simulink model "RasPiTCP_LedCtrl"  (R2018a)
settings: Solver=FixedStepAuto  StartTime=0.0  StopTime=inf  RelTol=1e-3  EnableMultiTasking=on
PreLoadFcn:
  | RasPiTcpConfig;
  | RasPiTcpDataType;
values from neighbouring files (symbols this model uses):
  LedInValidCommandMessage = 'Invalid Command'    [RasPiTcpConfig.m]
  LedOffMessage = "L.E.D is OFF   "    [RasPiTcpConfig.m]
  LedOnMessage = 'L.E.D is ON    '    [RasPiTcpConfig.m]
  TcpBufferInit = zeros(1,TcpBufferSize)    [RasPiTcpConfig.m]
undefined symbols (not defined in the file or in its folder): Green, led0, LedStatus
libraries: simulink x5, raspberrypilib x2, embdlinuxlib x2
settings Model: SimulationMode=external  Creator=swararag  LastModifiedBy=swararag
settings SolverCC: PositivePriorityOrder=on
settings OptimizationCC: EnhancedBackFolding=on  PassReuseOutputArgsAs=Individual arguments  MaxStackSize=64  OptimizeBlockOrder=speed  DifferentSizesBufferReuse=on  OptimizationCustomize=off
settings DebuggingCC: ParameterTunabilityLossMsg=error
settings HardwareCC: ProdBitPerPointer=32  ProdBitPerSizeT=32  ProdBitPerPtrDiffT=32  ProdLargestAtomicInteger=Long  ProdLargestAtomicFloat=Double  ProdWordSize=32  ProdHWDeviceType=ARM Compatible->ARM Cortex
settings SFSimCC: MATLABDynamicMemAlloc=off
settings RTWCC: SystemTargetFile=ert.tlc  HardwareBoard=Raspberry Pi  TLCOptions="-aInlineSetEventsForThisBaseRateFcn=TLC_FALSE -aSuppressMultiTaskScheduler=TLC_FALSE  -aRateBasedStepFcn=0"  TemplateMakefile=ert_default_tmf  GenerateReport=on  Toolchain=GNU GCC Raspberry Pi  BuildConfiguration=Faster Runs  IncludeHyperlinkInReport=on  LaunchReport=on  GenerateTraceInfo=on  GenerateTraceReport=on  GenerateTraceReportSl=on  GenerateTraceReportSf=on  GenerateTraceReportEml=on
settings CodeAppCC: ForceParamTrailComments=on  IgnoreCustomStorageClasses=off  OperatorAnnotations=on  SimulinkDataObjDesc=on  SFDataObjDesc=on  InsertBlockDesc=on
settings ERTTargetCC: SupportVariableSizeSignals=on  GenerateASAP2=on  ERTFilePackagingFormat=Compact

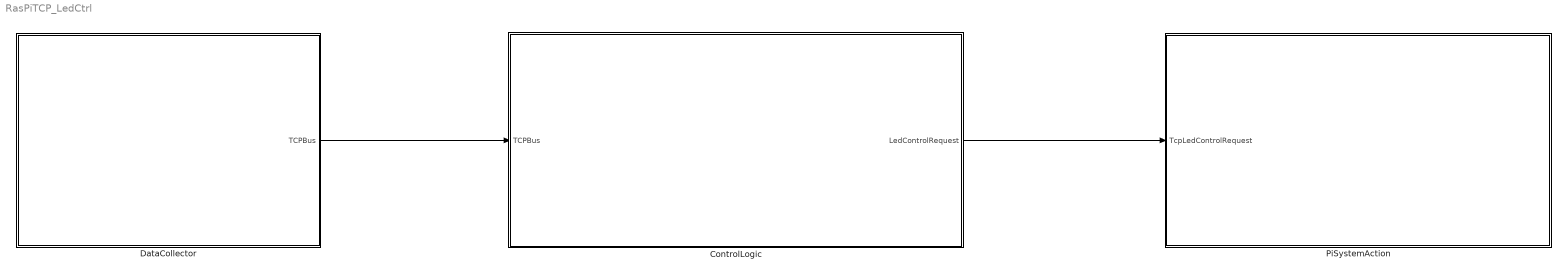
== system RasPiTCP_LedCtrl ==
  ControlLogic : Subsystem  Priority=1  TreatAsAtomicUnit=on
      settings: RTWFcnNameOpts=Use subsystem name
  DataCollector : Subsystem  Priority=0  TreatAsAtomicUnit=on
      settings: RTWFcnNameOpts=Use subsystem name
  PiSystemAction : Subsystem  Priority=2  TreatAsAtomicUnit=on
      settings: RTWFcnNameOpts=Use subsystem name  FunctionWithSeparateData=on
  wires:
  DataCollector/1(TCPBus) -> ControlLogic/1(TCPBus)
  ControlLogic/1(LedControlRequest) -> PiSystemAction/1(TcpLedControlRequest)

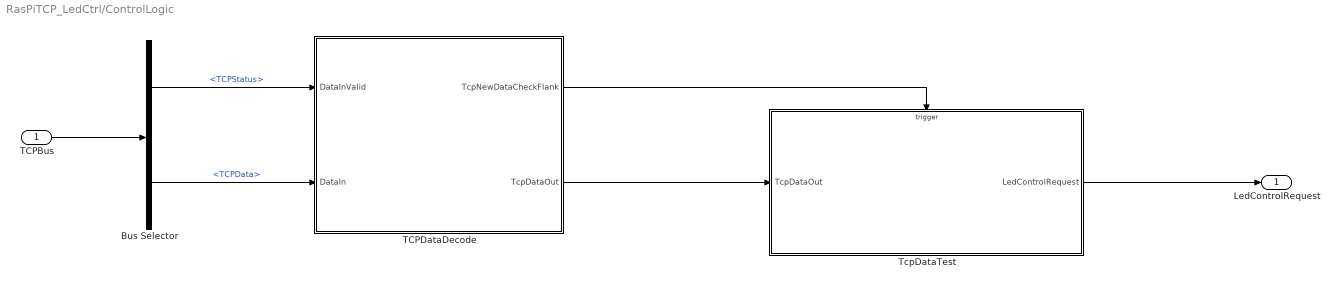
== system RasPiTCP_LedCtrl/ControlLogic ==
  TCPBus : Inport
  Bus Selector : BusSelector  OutputSignals=TCPStatus,TCPData
  TCPDataDecode : Subsystem  TreatAsAtomicUnit=on
  TcpDataTest : Subsystem
  LedControlRequest : Outport
  wires:
  TCPBus/1 -> Bus Selector/1
  Bus Selector/1 -> TCPDataDecode/1(DataInValid)  "<TCPStatus>"
  Bus Selector/2 -> TCPDataDecode/2(DataIn)  "<TCPData>"
  TCPDataDecode/2(TcpDataOut) -> TcpDataTest/1(TcpDataOut)
  TcpDataTest/1(LedControlRequest) -> LedControlRequest/1
  TCPDataDecode/1(TcpNewDataCheckFlank) -> TcpDataTest/Trigger

== system RasPiTCP_LedCtrl/DataCollector ==
  Bus Creator : BusCreator  Inputs=2
  Data Type Conversion : DataTypeConversion  OutDataTypeStr=boolean
  TCP/IP Receive : raspberrypilib/TCP//IP Receive  Mode_=Server  LocalServerPort_=TcpServerRxPort  RemoteAddr_=192.186.0.130  RemoteServerPort_=25001  DataType_=uint8  DataSize_=1  SampleTime_=0.05  SimulateUsing=Code generation  ClientPortBindingSelection_=off  ClientPortToBind_=35000  BlockingMode_=on  BlockTimeout_=TcpServerRxTimeOut
      settings: SourceProductName=Simulink Support Package for Raspberry Pi Hardware  SourceProductBaseCode=RASPPI
  TCPBus : Outport
  wires:
  TCP/IP Receive/2 -> Data Type Conversion/1
  Bus Creator/1 -> TCPBus/1
  Data Type Conversion/1 -> Bus Creator/2  "TCPStatus"
  TCP/IP Receive/1 -> Bus Creator/1  "TCPData"

== system RasPiTCP_LedCtrl/PiSystemAction ==
  TcpLedControlRequest : Inport
  Bus Selector : BusSelector  OutputSignals=LedControlRequestFlank,LedState
  TCPSend : Subsystem
      settings: RTWFcnNameOpts=Use subsystem name
  wires:
  TcpLedControlRequest/1 -> Bus Selector/1
  Bus Selector/2 -> TCPSend/1(LedStatus)  "<LedState>"
  Bus Selector/1 -> TCPSend/Trigger  "<LedControlRequestFlank>"

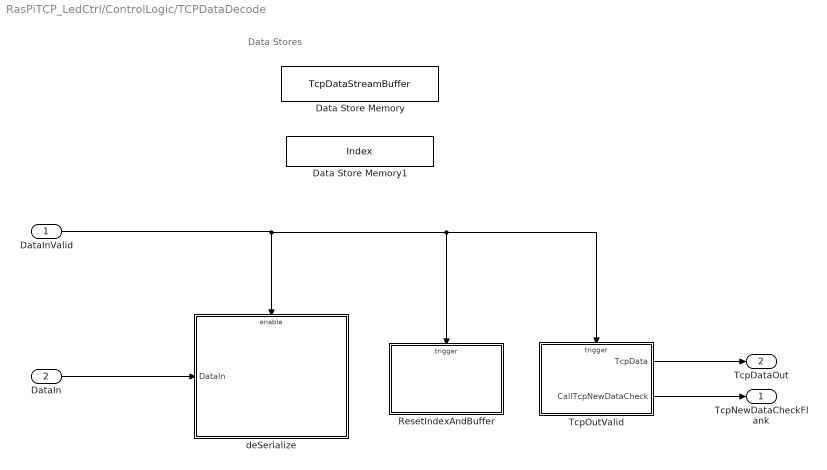
== system RasPiTCP_LedCtrl/ControlLogic/TCPDataDecode ==
  note: Data Stores
  DataInValid : Inport
  DataIn : Inport  Port=2
  Data Store Memory : DataStoreMemory  DataStoreName=TcpDataStreamBuffer  ReadBeforeWriteMsg=warning  WriteAfterWriteMsg=warning  WriteAfterReadMsg=warning  InitialValue=TcpBufferInit  ShowAdditionalParam=off  OutDataTypeStr=uint8
  Data Store Memory1 : DataStoreMemory  DataStoreName=Index  ReadBeforeWriteMsg=warning  WriteAfterWriteMsg=warning  WriteAfterReadMsg=warning  InitialValue=1  ShowAdditionalParam=off  OutDataTypeStr=uint8
  ResetIndexAndBuffer : Subsystem  Priority=0  TreatAsAtomicUnit=on
  TcpOutValid : Subsystem  Priority=1  TreatAsAtomicUnit=on
  deSerialize : Subsystem  Priority=0
  TcpNewDataCheckFlank : Outport
  TcpDataOut : Outport  Port=2
  wires:
  TcpOutValid/1(TcpData) -> TcpDataOut/1
  DataIn/1 -> deSerialize/1(DataIn)
  DataInValid/1 -> deSerialize/Enable, TcpOutValid/Trigger, ResetIndexAndBuffer/Trigger
  TcpOutValid/2(CallTcpNewDataCheck) -> TcpNewDataCheckFlank/1

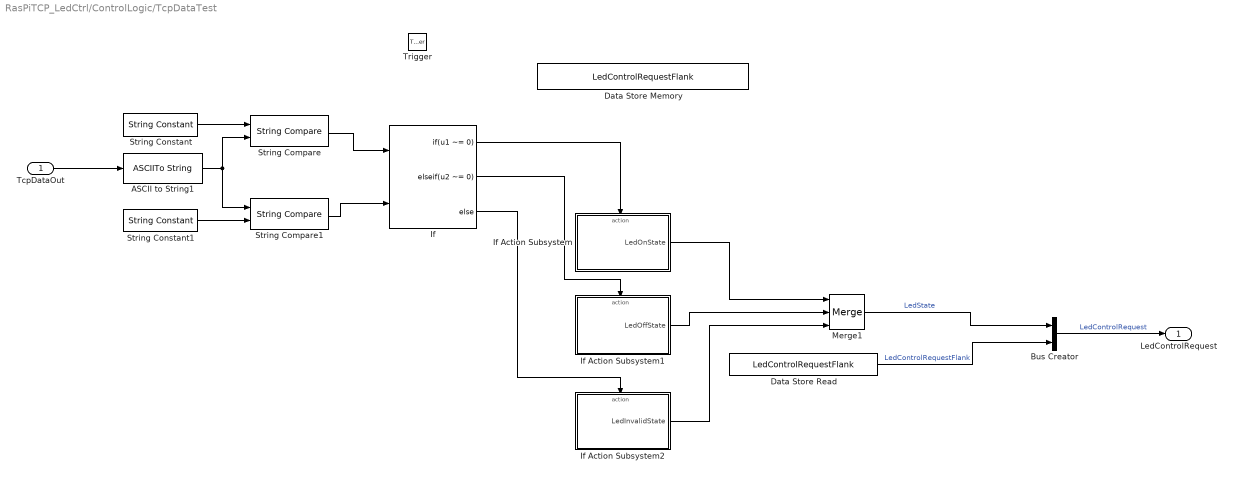
== system RasPiTCP_LedCtrl/ControlLogic/TcpDataTest ==
  TcpDataOut : Inport
  Trigger : TriggerPort  TriggerType=function-call  VariantControl=Variant  InitialTriggerSignalState=zero  PortDimensions=1
  ASCII to String1 : ASCIIToString
  Bus Creator : BusCreator  Inputs=2
  Data Store Memory : DataStoreMemory  DataStoreName=LedControlRequestFlank  ReadBeforeWriteMsg=warning  WriteAfterWriteMsg=warning  WriteAfterReadMsg=warning  InitialValue=1  ShowAdditionalParam=off  OutDataTypeStr=boolean
  Data Store Read : DataStoreRead  DataStoreName=LedControlRequestFlank
  If : If  NumInputs=2  IfExpression=u1 ~= 0  ElseIfExpressions=u2 ~= 0
  If Action Subsystem : Subsystem  TreatAsAtomicUnit=on
  If Action Subsystem1 : Subsystem  TreatAsAtomicUnit=on
  If Action Subsystem2 : Subsystem  TreatAsAtomicUnit=on
  Merge1 : Merge  Inputs=3  InitialOutput=LedStatus.OFF
  String Compare : StringCompare  CaseSensitive=off
  String Compare1 : StringCompare  CaseSensitive=off
  String Constant : StringConstant  String=LedOnText
  String Constant1 : StringConstant  String=LedOffText
  LedControlRequest : Outport
      settings: EnsureOutportIsVirtual=on
  wires:
  If/3 -> If Action Subsystem2/Action
  String Compare1/1 -> If/2
  ASCII to String1/1 -> String Compare1/1, String Compare/2
  If/2 -> If Action Subsystem1/Action
  If/1 -> If Action Subsystem/Action
  String Constant1/1 -> String Compare1/2
  String Constant/1 -> String Compare/1
  String Compare/1 -> If/1
  TcpDataOut/1 -> ASCII to String1/1
  If Action Subsystem2/1(LedInvalidState) -> Merge1/3
  If Action Subsystem1/1(LedOffState) -> Merge1/2
  If Action Subsystem/1(LedOnState) -> Merge1/1
  Merge1/1 -> Bus Creator/1  "LedState"
  Bus Creator/1 -> LedControlRequest/1  "LedControlRequest"
  Data Store Read/1 -> Bus Creator/2  "LedControlRequestFlank"

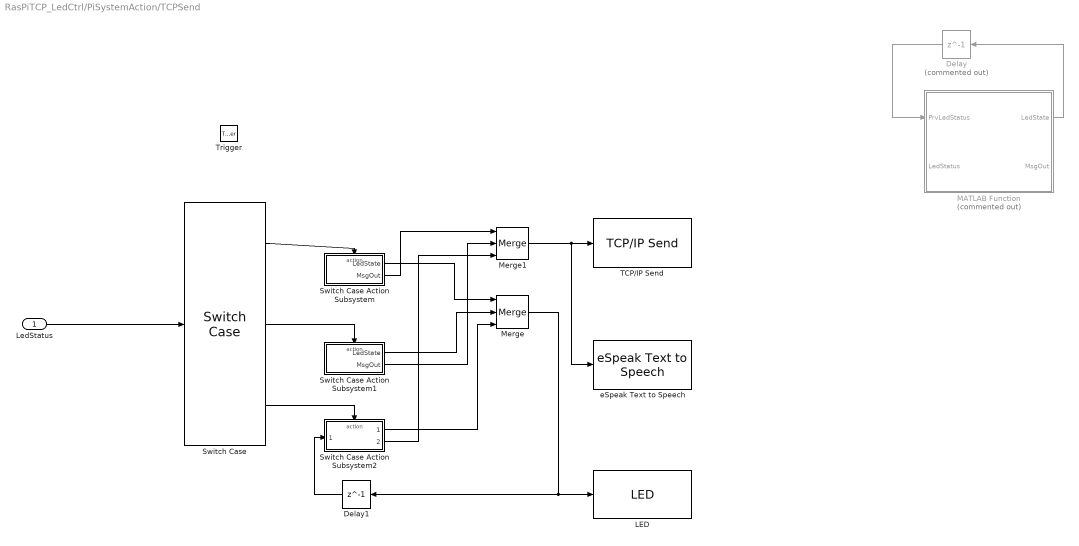
== system RasPiTCP_LedCtrl/PiSystemAction/TCPSend ==
  LedStatus : Inport  OutDataTypeStr=Enum: LedStatus
  Trigger : TriggerPort  TriggerType=either  VariantControl=Variant
  Delay : Delay  Commented=on  DelayLength=1  InitialCondition=false
  Delay1 : Delay  DelayLength=1  InitialCondition=false
  LED : embdlinuxlib/LED  board=Model B+  led=led0 (Green)  blockPlatform=Raspberry Pi
      settings: SourceProductName=Simulink Support Package for Raspberry Pi Hardware  SourceProductBaseCode=RASPPI
  MATLAB Function : MATLAB Function  Commented=on  TreatAsAtomicUnit=on
  Merge : Merge  Inputs=3  InitialOutput=false
  Merge1 : Merge  Inputs=3
  Switch Case : SwitchCase  CaseConditions={LedStatus.ON, LedStatus.OFF}
  Switch Case Action Subsystem : Subsystem  TreatAsAtomicUnit=on
  Switch Case Action Subsystem1 : Subsystem  TreatAsAtomicUnit=on
  Switch Case Action Subsystem2 : Subsystem  TreatAsAtomicUnit=on
  TCP/IP Send : raspberrypilib/TCP//IP Send  Mode_=Server  LocalServerPort_=TcpServerTxPort  RemoteAddr_=192.168.0.117  RemoteServerPort_=25000  SimulateUsing=Code generation  ClientPortBindingSelection_=off  ClientPortToBind_=35000  BlockingMode_=on  BlockTimeout_=TcpServerTxTimeOut
      settings: SourceProductName=Simulink Support Package for Raspberry Pi Hardware  SourceProductBaseCode=RASPPI
  eSpeak Text to Speech : embdlinuxlib/eSpeak Text to Speech  blockPlatform=Raspberry Pi
      settings: SourceProductName=Simulink Support Package for Raspberry Pi Hardware  SourceProductBaseCode=RASPPI
  wires:
  MATLAB Function/1(LedState) -> Delay/1
  Switch Case/1 -> Switch Case Action Subsystem/Action
  Switch Case/2 -> Switch Case Action Subsystem1/Action
  Switch Case Action Subsystem/1(LedState) -> Merge/1
  Switch Case Action Subsystem1/1(LedState) -> Merge/2
  LedStatus/1 -> Switch Case/1
  Delay/1 -> MATLAB Function/1(PrvLedStatus)
  Switch Case/3 -> Switch Case Action Subsystem2/Action
  Switch Case Action Subsystem2/1(LedState) -> Merge/3
  Merge/1 -> Delay1/1, LED/1
  Delay1/1 -> Switch Case Action Subsystem2/1(PrvState)
  Merge1/1 -> eSpeak Text to Speech/1, TCP/IP Send/1
  Switch Case Action Subsystem2/2(MsgOut) -> Merge1/3
  Switch Case Action Subsystem1/2(MsgOut) -> Merge1/2
  Switch Case Action Subsystem/2(MsgOut) -> Merge1/1

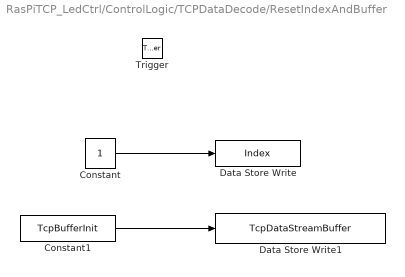
== system RasPiTCP_LedCtrl/ControlLogic/TCPDataDecode/ResetIndexAndBuffer ==
  Trigger : TriggerPort  VariantControl=Variant  InitialTriggerSignalState=zero  PortDimensions=1
  Constant : Constant  OutDataTypeStr=uint8
  Constant1 : Constant  Value=TcpBufferInit  OutDataTypeStr=uint8
  Data Store Write : DataStoreWrite  DataStoreName=Index
  Data Store Write1 : DataStoreWrite  DataStoreName=TcpDataStreamBuffer
  wires:
  Constant/1 -> Data Store Write/1
  Constant1/1 -> Data Store Write1/1

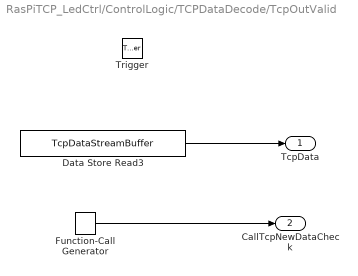
== system RasPiTCP_LedCtrl/ControlLogic/TCPDataDecode/TcpOutValid ==
  Trigger : TriggerPort  TriggerType=falling  VariantControl=Variant  InitialTriggerSignalState=zero  PortDimensions=1
  Data Store Read3 : DataStoreRead  DataStoreName=TcpDataStreamBuffer
  Function-Call Generator : simulink/Ports & Subsystems/Function-Call Generator  sample_time=-1  numberOfIterations=1
  TcpData : Outport
  CallTcpNewDataCheck : Outport  Port=2
  wires:
  Data Store Read3/1 -> TcpData/1
  Function-Call Generator/1 -> CallTcpNewDataCheck/1

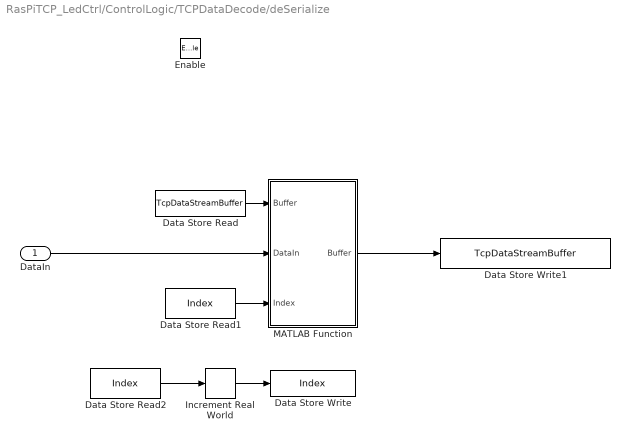
== system RasPiTCP_LedCtrl/ControlLogic/TCPDataDecode/deSerialize ==
  DataIn : Inport
  Enable : EnablePort  PropagateVarSize=During execution
  Data Store Read : DataStoreRead  DataStoreName=TcpDataStreamBuffer
  Data Store Read1 : DataStoreRead  DataStoreName=Index
  Data Store Read2 : DataStoreRead  Priority=8  DataStoreName=Index
  Data Store Write : DataStoreWrite  DataStoreName=Index
  Data Store Write1 : DataStoreWrite  DataStoreName=TcpDataStreamBuffer
  Increment Real World : simulink/Additional Math & Discrete/Additional Math: Increment - Decrement/Increment Real World
      settings: SourceProductName=Simulink  SourceProductBaseCode=SL
  MATLAB Function : MATLAB Function  Priority=1  TreatAsAtomicUnit=on
  wires:
  DataIn/1 -> MATLAB Function/2(DataIn)
  MATLAB Function/1(Buffer) -> Data Store Write1/1
  Data Store Read/1 -> MATLAB Function/1("Buffer ")
  Data Store Read1/1 -> MATLAB Function/3(Index)
  Increment Real World/1 -> Data Store Write/1
  Data Store Read2/1 -> Increment Real World/1

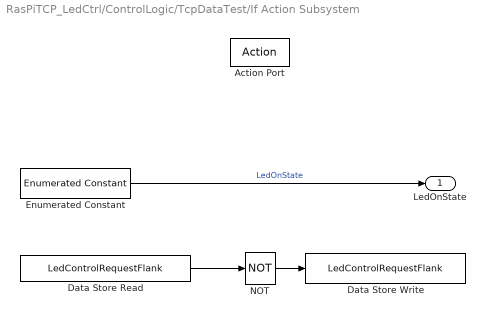
== system RasPiTCP_LedCtrl/ControlLogic/TcpDataTest/If Action Subsystem ==
  Action Port : ActionPort  ActionType=then
  Data Store Read : DataStoreRead  DataStoreName=LedControlRequestFlank
  Data Store Write : DataStoreWrite  DataStoreName=LedControlRequestFlank
  Enumerated Constant : simulink/Sources/Enumerated Constant  OutDataTypeStr=Enum: LedStatus  Value=LedStatus.ON  SampleTime=inf
      settings: SourceProductName=Simulink
  NOT : Logic  Operator=NOT  IconShape=distinctive  AllPortsSameDT=off  OutDataTypeStr=boolean
  LedOnState : Outport
  wires:
  Enumerated Constant/1 -> LedOnState/1  "LedOnState"
  Data Store Read/1 -> NOT/1
  NOT/1 -> Data Store Write/1

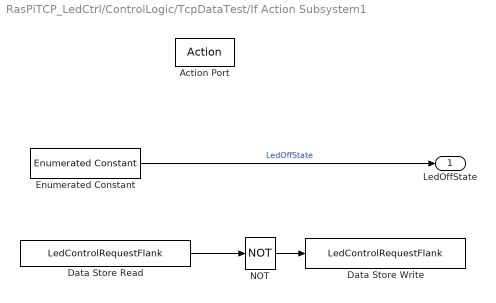
== system RasPiTCP_LedCtrl/ControlLogic/TcpDataTest/If Action Subsystem1 ==
  Action Port : ActionPort  ActionType=elseif
  Data Store Read : DataStoreRead  DataStoreName=LedControlRequestFlank
  Data Store Write : DataStoreWrite  DataStoreName=LedControlRequestFlank
  Enumerated Constant : simulink/Sources/Enumerated Constant  OutDataTypeStr=Enum: LedStatus  Value=LedStatus.OFF  SampleTime=inf
      settings: SourceProductName=Simulink
  NOT : Logic  Operator=NOT  IconShape=distinctive  AllPortsSameDT=off  OutDataTypeStr=boolean
  LedOffState : Outport
  wires:
  Enumerated Constant/1 -> LedOffState/1  "LedOffState"
  Data Store Read/1 -> NOT/1
  NOT/1 -> Data Store Write/1

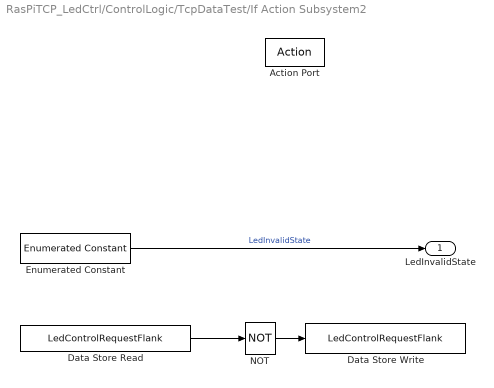
== system RasPiTCP_LedCtrl/ControlLogic/TcpDataTest/If Action Subsystem2 ==
  Action Port : ActionPort  ActionType=else
  Data Store Read : DataStoreRead  DataStoreName=LedControlRequestFlank
  Data Store Write : DataStoreWrite  DataStoreName=LedControlRequestFlank
  Enumerated Constant : simulink/Sources/Enumerated Constant  OutDataTypeStr=Enum: LedStatus  Value=LedStatus.INVALID  SampleTime=inf
      settings: SourceProductName=Simulink
  NOT : Logic  Operator=NOT  IconShape=distinctive  AllPortsSameDT=off  OutDataTypeStr=boolean
  LedInvalidState : Outport
  wires:
  Enumerated Constant/1 -> LedInvalidState/1  "LedInvalidState"
  Data Store Read/1 -> NOT/1
  NOT/1 -> Data Store Write/1

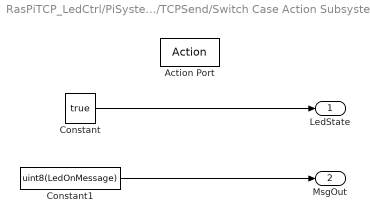
== system RasPiTCP_LedCtrl/PiSystemAction/TCPSend/Switch Case Action Subsystem ==
  Action Port : ActionPort  ActionType=case
  Constant : Constant  Value=true  OutDataTypeStr=boolean
  Constant1 : Constant  Value=uint8(LedOnMessage)  OutDataTypeStr=uint8
  LedState : Outport
  MsgOut : Outport  Port=2
  wires:
  Constant/1 -> LedState/1
  Constant1/1 -> MsgOut/1

== system RasPiTCP_LedCtrl/PiSystemAction/TCPSend/Switch Case Action Subsystem1 ==
  Action Port : ActionPort  ActionType=case
  Constant : Constant  Value=false  OutDataTypeStr=boolean
  Constant1 : Constant  Value=uint8(LedOffMessage)  OutDataTypeStr=uint8
  LedState : Outport
  MsgOut : Outport  Port=2
  wires:
  Constant/1 -> LedState/1
  Constant1/1 -> MsgOut/1

== system RasPiTCP_LedCtrl/PiSystemAction/TCPSend/Switch Case Action Subsystem2 ==
  PrvState : Inport
  Action Port : ActionPort  ActionType=default
  Constant1 : Constant  Value=uint8(LedInValidCommandMessage)  OutDataTypeStr=uint8
  LedState : Outport
  MsgOut : Outport  Port=2
  wires:
  PrvState/1 -> LedState/1
  Constant1/1 -> MsgOut/1

== matlab function RasPiTCP_LedCtrl/ControlLogic/TCPDataDecode/deSerialize/MATLAB Function ==
  data: Buffer input; DataIn input; Index input; Buffer output
function Buffer =fcn(Buffer,DataIn,Index)


Buffer(Index)=DataIn;


end

== matlab function RasPiTCP_LedCtrl/PiSystemAction/TCPSend/MATLAB Function ==
  data: PrvLedStatus input; LedStatus input; LedState output; MsgOut output
function [LedState,MsgOut]= fcn(PrvLedStatus,LedStatus)

switch LedStatus
   case OFF
        LedState = false; 
        MsgOut = uint8('L.E.D is OFF   ');
   case 1
        LedState = true;
        MsgOut = uint8('L.E.D is ON    ');
    otherwise
        LedState=PrvLedStatus;
        MsgOut = uint8('Invalid Command');
end


end
